simulink model "stabil"  (R2022b)
settings: Solver=VariableStepAuto  StartTime=0.0  StopTime=100  RelTol=1e-3
values from neighbouring files (symbols this model uses):
  k = ki(i)    [regPI.m]    (also in regulator.m = kp(i))
settings Model: Creator=wojna  LastModifiedBy=wojna

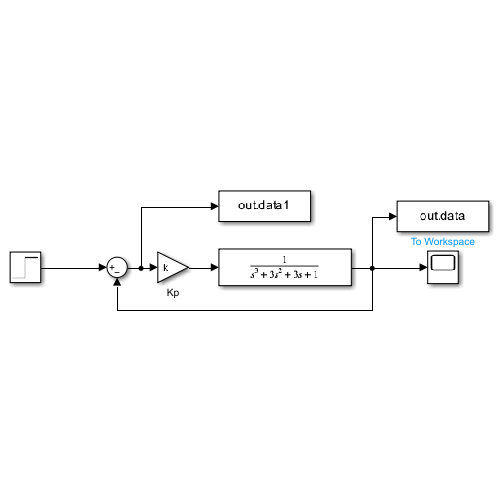
[thumbnail: Simulink's stored preview of the top-level diagram]
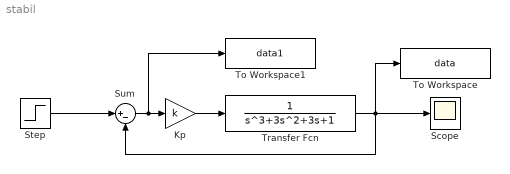
== system stabil ==
  Kp : Gain  Gain=k
  Scope : Scope
  Step : Step  SampleTime=0
  Sum : Sum  Inputs=|+-
  To Workspace : ToWorkspace  VariableName=data  SaveFormat=Timeseries  SampleTime=-1
  To Workspace1 : ToWorkspace  VariableName=data1  SaveFormat=Timeseries  SampleTime=-1
  Transfer Fcn : TransferFcn  Denominator=[1 3 3 1]
  wires:
  Step/1 -> Sum/1
  Sum/1 -> To Workspace1/1, Kp/1
  Kp/1 -> Transfer Fcn/1
  Transfer Fcn/1 -> To Workspace/1, Sum/2, Scope/1
